simulink model "func6"  (R2016a)
settings: Solver=VariableStepAuto  StartTime=0.0  StopTime=10.0  RelTol=1e-3
libraries: ModelComposer x4, templatized_input_6_lib x2
settings Model: Creator=abehbood  LastModifiedBy=abehbood
settings GRTTargetCC: GeneratePreprocessorConditionals=Use local settings

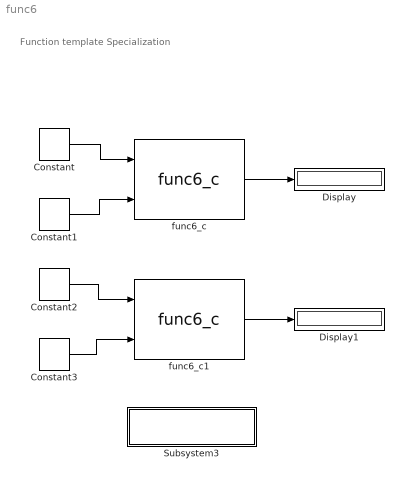
== system func6 ==
  note: Function template Specialization
  Constant : ModelComposer/Constant  Value=1  SampleTime=1  OutDataType=boolean  TypeExp=''  Signedness=Signed  WordLength=16  FractionalLength=0  RoundingMode=Truncation to minus infinity  OverflowMode=Wrap around
  Constant1 : ModelComposer/Constant  Value=0  SampleTime=1  OutDataType=boolean  TypeExp=''  Signedness=Signed  WordLength=16  FractionalLength=0  RoundingMode=Truncation to minus infinity  OverflowMode=Wrap around
  Constant2 : ModelComposer/Constant  Value=12  SampleTime=1  OutDataType=uint8  TypeExp=''  Signedness=Signed  WordLength=16  FractionalLength=0  RoundingMode=Truncation to minus infinity  OverflowMode=Wrap around
  Constant3 : ModelComposer/Constant  Value=20  SampleTime=1  OutDataType=uint8  TypeExp=''  Signedness=Signed  WordLength=16  FractionalLength=0  RoundingMode=Truncation to minus infinity  OverflowMode=Wrap around
  Display : Display
  Display1 : Display
  Subsystem3 : Subsystem
      settings: OpenFcn=xmcOpenFileEx
      mask Display: disp(sprintf('Double Click to open\nthe main header file'))
  func6_c : templatized_input_6_lib/func6_c  LibraryFunction=func6_c  IncludeFiles={'func6_c.h'}  SourceFiles={}  IncludeDirectories={'$XILINX_VIVADO/include'}  TemplateParams={'typename T'}  FunctionParamTypes={xmcDataType('T'); xmcDataType('T'); xmcDataType('T')}  FunctionParamPassbys={0.000000000000000000e+00; 0.000000000000000000e+00; 0.000000000000000000e+00}  FunctionParamDimensions={'1'; '1'; '1'}  FunctionParamNames={'return'; 'x'; 'y'}  FunctionParamDir={2.000000000000000000e+00; 1.000000000000000000e+00; 1.000000000000000000e+00}  FunctionParamSupportsStreaming={false; false; false}  BufferDepth={'0'}  FunctionParamValues={'0'; '0'; '0'}  ThroughputFactors={''}
  func6_c1 : templatized_input_6_lib/func6_c  LibraryFunction=func6_c  IncludeFiles={'func6_c.h'}  SourceFiles={}  IncludeDirectories={'$XILINX_VIVADO/include'}  TemplateParams={'typename T'}  FunctionParamTypes={xmcDataType('T'); xmcDataType('T'); xmcDataType('T')}  FunctionParamPassbys={0.000000000000000000e+00; 0.000000000000000000e+00; 0.000000000000000000e+00}  FunctionParamDimensions={'1'; '1'; '1'}  FunctionParamNames={'return'; 'x'; 'y'}  FunctionParamDir={2.000000000000000000e+00; 1.000000000000000000e+00; 1.000000000000000000e+00}  FunctionParamSupportsStreaming={false; false; false}  BufferDepth={'0'}  FunctionParamValues={'0'; '0'; '0'}  ThroughputFactors={''}
  wires:
  func6_c/1 -> Display/1
  Constant1/1 -> func6_c/2
  Constant/1 -> func6_c/1
  Constant2/1 -> func6_c1/1
  Constant3/1 -> func6_c1/2
  func6_c1/1 -> Display1/1

== system func6/Subsystem3 ==
